simulink model "YAW_usporedba"  (R2020b)
settings: Solver=VariableStepAuto  StartTime=0.0  StopTime=10.0  RelTol=1e-3
undefined symbols (not defined in the file): k_y2, wn_y2, zeta_y2
settings Model: Creator=Ivan  LastModifiedBy=Ivan

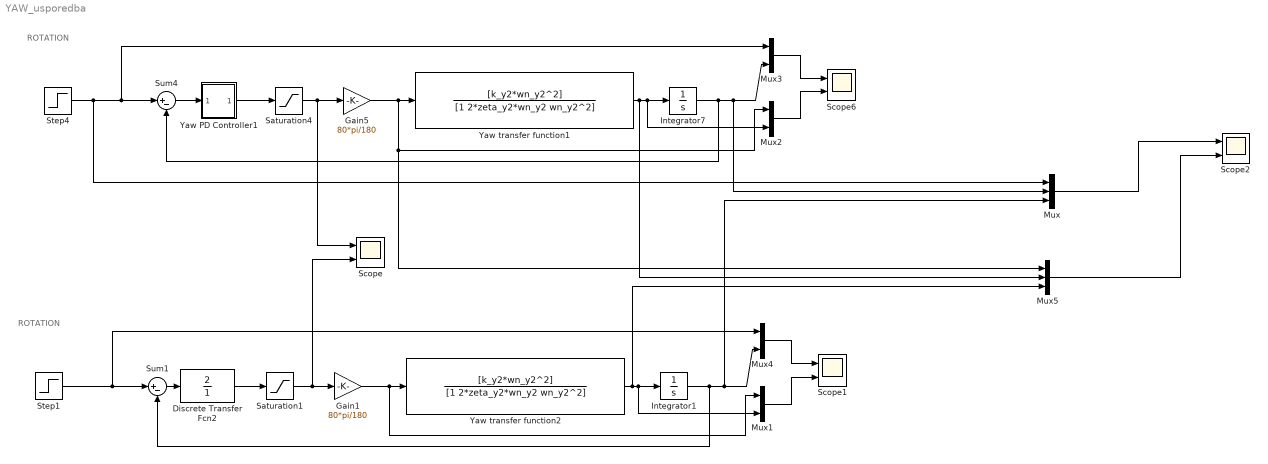
== system YAW_usporedba ==
  note: ROTATION
  note: ROTATION
  Discrete Transfer Fcn2 : DiscreteTransferFcn  Numerator=[2]  Denominator=[1]  SampleTime=0.1
  Gain1 : Gain  Gain=80*pi/180
  Gain5 : Gain  Gain=80*pi/180
  Integrator1 : Integrator
  Integrator7 : Integrator
  Mux : Mux  Inputs=3
  Mux{1..4} (4 alike) : Mux  Inputs=2
  Mux5 : Mux  Inputs=3
  Saturation1 : Saturate  UpperLimit=1  LowerLimit=-1
  Saturation4 : Saturate  UpperLimit=1  LowerLimit=-1
  Scope{,1..2,6} (4 alike) : Scope  NumInputPorts=2
  Step1 : Step  Time=0  After=pi/4  SampleTime=0
  Step4 : Step  Time=0  After=pi/4  SampleTime=0
  Sum1 : Sum  Inputs=|+-
  Sum4 : Sum  Inputs=|+-
  Yaw PD Controller1 : Subsystem
  Yaw transfer function1 : TransferFcn  Numerator=[k_y2*wn_y2^2]  Denominator=[1 2*zeta_y2*wn_y2 wn_y2^2]
  Yaw transfer function2 : TransferFcn  Numerator=[k_y2*wn_y2^2]  Denominator=[1 2*zeta_y2*wn_y2 wn_y2^2]
  wires:
  Mux2/1 -> Scope6/2
  Step4/1 -> Mux/1, Mux3/1, Sum4/1
  Mux3/1 -> Scope6/1
  Integrator7/1 -> Sum4/2, Mux/2, Mux3/2
  Gain5/1 -> Mux5/1, Mux2/1, Yaw transfer function1/1
  Saturation4/1 -> Scope/1, Gain5/1
  Yaw transfer function1/1 -> Mux5/2, Mux2/2, Integrator7/1
  Yaw PD Controller1/1("  ") -> Saturation4/1
  Sum4/1 -> Yaw PD Controller1/1(" ")
  Mux1/1 -> Scope1/2
  Sum1/1 -> Discrete Transfer Fcn2/1
  Mux4/1 -> Scope1/1
  Discrete Transfer Fcn2/1 -> Saturation1/1
  Integrator1/1 -> Sum1/2, Mux/3, Mux4/2
  Step1/1 -> Mux4/1, Sum1/1
  Yaw transfer function2/1 -> Mux5/3, Mux1/2, Integrator1/1
  Saturation1/1 -> Scope/2, Gain1/1
  Gain1/1 -> Mux1/1, Yaw transfer function2/1
  Mux/1 -> Scope2/1
  Mux5/1 -> Scope2/2

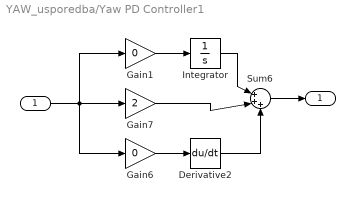
== system YAW_usporedba/Yaw PD Controller1 ==
  " " : Inport
  Derivative2 : Derivative
  Gain1 : Gain  Gain=0
  Gain6 : Gain  Gain=0
  Gain7 : Gain  Gain=2
  Integrator : Integrator
  Sum6 : Sum  Inputs=|+++
  "  " : Outport
  wires:
  Sum6/1 -> "  "/1
  Derivative2/1 -> Sum6/3
  " "/1 -> Gain1/1, Gain7/1, Gain6/1
  Gain6/1 -> Derivative2/1
  Gain7/1 -> Sum6/2
  Integrator/1 -> Sum6/1
  Gain1/1 -> Integrator/1
